simulink model "observador"  (R2023a)
settings: Solver=ode4  StartTime=0.0  StopTime=5  FixedStep=0.01  RelTol=1e-3
values from neighbouring files (symbols this model uses):
  A = [-6 -3 -2;22 5 10;-12 0 -7]    [eje4_par3.m]    (also in ejer1_par3.m = [9 -28 -40; 10 -28 -35;-4 11 12]; ejer2_par3.m = [8 -12 4;3 -4 1;-21 30 -11]; ejer3_par3.m = [101 -6 56;-121 4 -65;-208 12 -115]; ejer5_par3.m = [-16 -25 25; -7 -12 9;-17 -26 23])
  B = [-8;11;9]    [eje4_par3.m]    (also in ejer2_par3.m = [6;-6;-32]; ejer3_par3.m = [-1;2;2]; ejer5_par3.m = [-2;0;-2])
  C = [50 20 22]    [eje4_par3.m]    (also in ejer3_par3.m = [-108 6 -58])
  L = place(A',C',lamObs')'    [eje4_par3.m]    (also in ejer3_par3.m = place(A',C',lamR')')
  x0 = [3;-9;8]    [eje4_par3.m]    (also in ejer2_par3.m = [-3,9,-10]; ejer3_par3.m = [-10;-7;-7])
  x0h = [0;0;0]    [eje4_par3.m]    (also in ejer3_par3.m)
settings Model: Creator=itzel  LastModifiedBy=userh
settings OptimizationCC: ReuseModelBlockBuffer=off

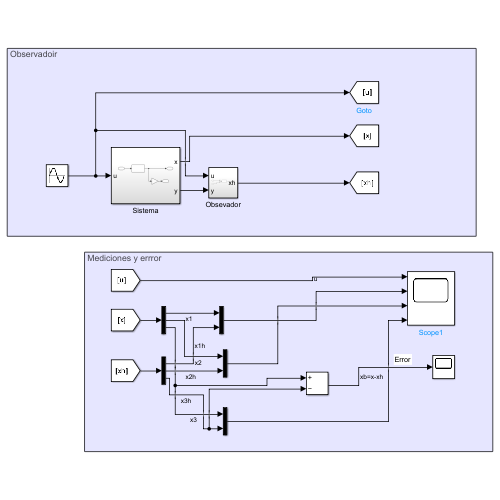
[thumbnail: Simulink's stored preview of the top-level diagram]
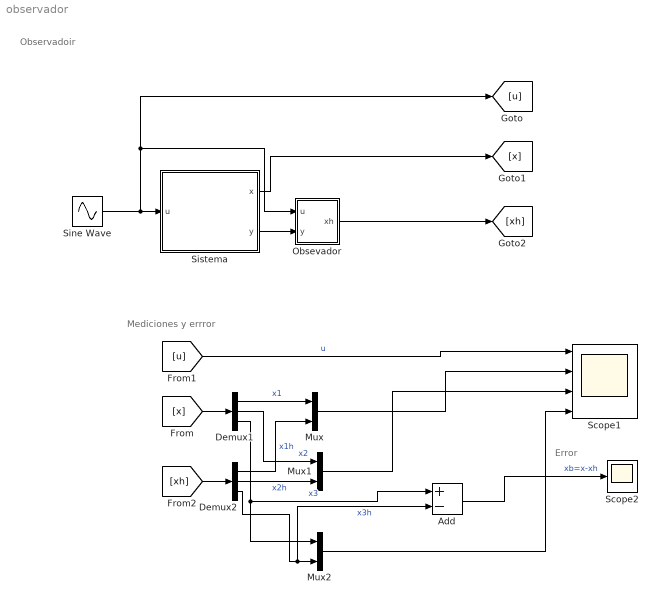
== system observador ==
  note: Mediciones y errror
  note: Observadoir
  note: Error
  Add : Sum  Inputs=+-
  Demux1 : Demux  Outputs=3
  Demux2 : Demux  Outputs=3
  Mux : Mux  Inputs=2
  Mux1 : Mux  Inputs=2
  Mux2 : Mux  Inputs=2
  Obsevador : Subsystem
  Scope1 : Scope  NumInputPorts=4
  Scope2 : Scope
  Sine Wave : Sin  Amplitude=4  Frequency=2  SampleTime=0
  Sistema : Subsystem
  wires:
  Mux2/1 -> Scope1/4
  Mux1/1 -> Scope1/3
  Demux2/1 -> Mux/2  "x1h"
  [x] -> Demux1/1
  Demux2/2 -> Mux1/2  "x2h"
  Demux1/2 -> Mux1/1  "x2"
  [u] -> Scope1/1  "u"
  Sistema/1(x) -> [x]
  Sine Wave/1 -> [u], Obsevador/1(u), Sistema/1(u)
  Demux1/1 -> Mux/1  "x1"
  [xh] -> Demux2/1
  Obsevador/1(xh) -> [xh]
  Add/1 -> Scope2/1  "xb=x-xh"
  Sistema/2(y) -> Obsevador/2(y)
  Demux1/3 -> Add/1, Mux2/1  "x3"
  Mux/1 -> Scope1/2
  Demux2/3 -> Add/2, Mux2/2  "x3h"

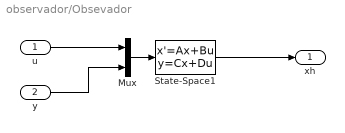
== system observador/Obsevador ==
  u : Inport
  y : Inport  Port=2
  Mux : Mux  Inputs=2
  State-Space1 : StateSpace  A=A-L*C  B=[B,L]  C=eye(3)  D=zeros(3,2)  InitialCondition=x0h  ParameterTunability=Unconstrained  AllowTunableDMatrix=on
  xh : Outport
  wires:
  Mux/1 -> State-Space1/1
  u/1 -> Mux/1
  State-Space1/1 -> xh/1
  y/1 -> Mux/2

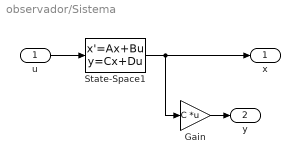
== system observador/Sistema ==
  u : Inport
  Gain : Gain  Gain=C  Multiplication=Matrix(K*u)
  State-Space1 : StateSpace  A=A  B=B  C=eye(3)  D=zeros(3,1)  InitialCondition=x0
  x : Outport
  y : Outport  Port=2
  wires:
  Gain/1 -> y/1
  State-Space1/1 -> x/1, Gain/1
  u/1 -> State-Space1/1
